simulink model "reverberancia"  (Simulink 7.2)
settings: Solver=ode45  StartTime=0.0  StopTime=8  RelTol=1e-3
libraries: dspsigops x1, dspsrcs4 x1, dspsnks4 x1
settings Model: Creator=Gus  LastModifiedBy=Gus
settings SimEventsCC: propLogEventsScheduled=0  propLogEventsExecuted=0  propLogDepartureEvents=0  propDisplayEventCalendar=0  propDiagAttribOutput=1  propDiagFcnCallOutput=1  propDiagStatOutput=0

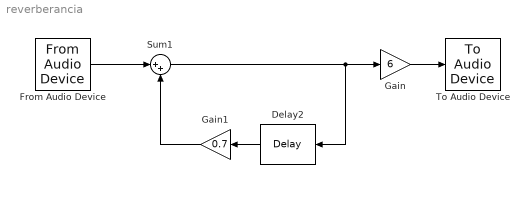
== system reverberancia ==
  Delay2 : dspsigops/Delay  Orientation=left  dly_unit=Samples  delay=44100*0.1  ic_detail=off  dif_ic_for_ch=off  dif_ic_for_dly=off  ic=0  reset_popup=None
  From Audio Device : dspsrcs4/From Audio Device  DialogController=dspDDGCreate  DialogControllerArgs=DataTag0  deviceName=Default  numChannels=1  sampleRate=44100  deviceDatatype=Determine from output data type  autoBufferSize=on  bufferSize=4096  queueDuration=1.0  frameSize=1024  outputDatatype=single
  Gain : Gain  Gain=6  ParameterDataType=sfix(16)  ParameterScaling=2^0  OutDataType=sfix(16)  OutScaling=2^0
  Gain1 : Gain  Orientation=left  Gain=0.7  ParameterDataType=sfix(16)  ParameterScaling=2^0  OutDataType=sfix(16)  OutScaling=2^0
  Sum1 : Sum  Inputs=|++  OutDataType=sfix(16)  OutScaling=2^0
  To Audio Device : dspsnks4/To Audio Device  DialogController=dspDDGCreate  DialogControllerArgs=DataTag1  deviceName=Default  inheritSampleRate=on  sampleRate=44100  deviceDatatype=Determine from input data type  autoBufferSize=on  bufferSize=4096  queueDuration=1.0
  wires:
  Gain/1 -> To Audio Device/1
  Sum1/1 -> Delay2/1, Gain/1
  Delay2/1 -> Gain1/1
  Gain1/1 -> Sum1/2
  From Audio Device/1 -> Sum1/1
